simulink model "fsm_model_test"  (Simulink 8.0)
settings: Solver=ode3  StartTime=0.0  StopTime=inf  FixedStep=0.0001  RelTol=1e-3
libraries: simulink x1
settings Model: RequirementInfo={} %GIDa_df0a3179_6454_4361_a9b2_385228527c42  Creator=caster  LastModifiedBy=caster
settings DebuggingCC: ModelReferenceSymbolNameMessage=none

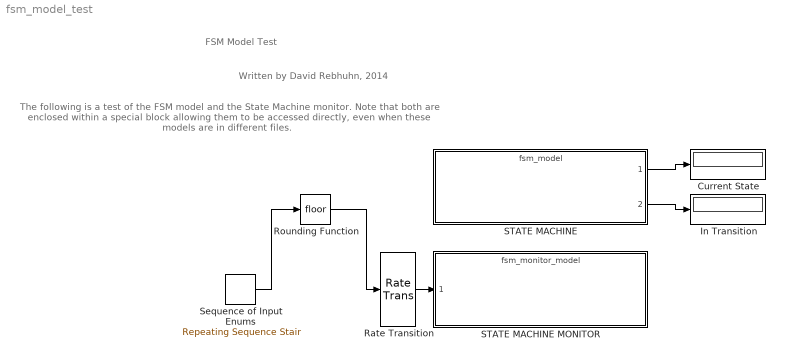
== system fsm_model_test ==
  note: Written by David Rebhuhn, 2014
  note: The following is a test of the FSM model and the State Machine monitor.
      | Note that both are enclosed within a special block allowing them to be
      | accessed directly, even when these models are in different files.
  note: FSM Model Test
  Current State : Display
  In Transition : Display
  Rate Transition : RateTransition
  Rounding Function : Rounding
  STATE MACHINE : ModelReference  ModelNameDialog=fsm_model  SimulationMode=Normal  ModelReferenceVersion=1.8  CopyOfModelName=fsm_model  DefaultDataLogging=on
  STATE MACHINE MONITOR : ModelReference  ModelNameDialog=fsm_monitor_model  SimulationMode=Normal  ModelReferenceVersion=1.6  CopyOfModelName=fsm_monitor_model  DefaultDataLogging=on
  Sequence of Input Enums : simulink/Sources/Repeating Sequence Stair  OutValues=[1 2 3 4 5 2 7]  tsamp=4  OutMin=[]  OutMax=[]  OutDataTypeStr=double  OutputDataTypeScalingMode=double  OutDataType=fixdt(0,8)  ConRadixGroup=Best Precision: Vector-wise  OutScaling=2^-12
  wires:
  Sequence of Input Enums/1 -> Rounding Function/1
  STATE MACHINE/2 -> In Transition/1
  STATE MACHINE/1 -> Current State/1
  Rounding Function/1 -> Rate Transition/1
  Rate Transition/1 -> STATE MACHINE MONITOR/1
